simulink model "rle7"  (R2025b)
settings: Solver=FixedStepAuto  StartTime=0.0  StopTime=t_stop  FixedStep=1e-3  MaxStep=1e-3  RelTol=1e-3
values from neighbouring files (symbols this model uses):
  den_ac = [1, 2.35, -5.31, 0.184, -0.041]    [indf.m]    (also in indf_v8.m; rlelog5.m = [1 0.8608 5.3159942 0.108928 0.0529])
  Kp = 1    [Comparisons_of_Examples_OLOP_Jump_Frequency.m]    (also in LimitCycleAnalysisbyNIDF_GUI.m = appData.Kp.Value; OLOP_GUI.m = KpEdit.Value; PIO_LimitCycleApp.m = Kp_vec(j); ashkenas.m)
  num_ac = -10.524 * [1, 1.6, 0.059, 0]    [indf.m]    (also in indf_v8.m; rlelog5.m = [3.476 3.1708072 0.0896237936])
  R = 15    [Comparisons_of_Examples_OLOP_Jump_Frequency.m]    (also in Fig16_OLOP_Nichols.m = 5; LimitCycleAnalysisbyNIDF_GUI.m = appData.R.Value; OLOP_GUI.m = REdit.Value; Olop_nichols_fig16.m = 5)
settings Model: Creator=t0900  LastModifiedBy=t0900

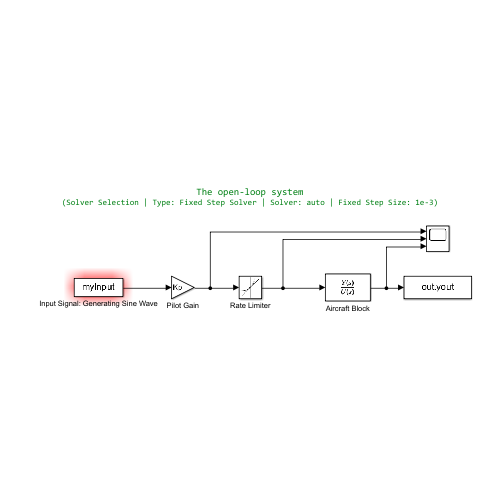
[thumbnail: Simulink's stored preview of the top-level diagram]
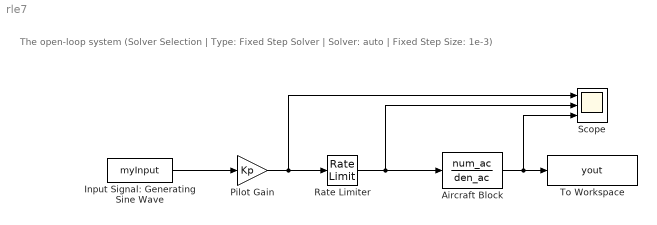
== system rle7 ==
  note: The open-loop system
      | (Solver Selection | Type: Fixed Step Solver | Solver: auto | Fixed Step Size: 1e-3)
  Aircraft Block : TransferFcn  Numerator=num_ac  Denominator=den_ac
  Input Signal: Generating Sine Wave : FromWorkspace  VariableName=myInput
  Pilot Gain : Gain  Gain=Kp
  Rate Limiter : RateLimiter  RisingSlewLimit=R  FallingSlewLimit=-R
  Scope : Scope  NumInputPorts=3
      settings: ActiveDisplayYMinimum=-4.3749954725549358  ActiveDisplayYMaximum=4.3749951589791722
  To Workspace : ToWorkspace  VariableName=yout  SampleTime=-1
  wires:
  Rate Limiter/1 -> Scope/2, Aircraft Block/1
  Input Signal: Generating Sine Wave/1 -> Pilot Gain/1
  Pilot Gain/1 -> Scope/1, Rate Limiter/1
  Aircraft Block/1 -> Scope/3, To Workspace/1
